simulink model "paper1"  (Simulink 6.0)
settings: Solver=ode45  StartTime=0.0  StopTime=30.0  RelTol=1e-3
values from neighbouring files (symbols this model uses):
  bp = 0.0    (= 0)    [paper1_data.m]
  bt = 0.8    [paper1_data.m]
  En = 1.0    (= 1)    [paper1_data.m]
  Eqh = 0.5    [paper1_data.m]
  Ey = 1.0    (= 1)    [paper1_data.m]
  Ta = 5    [paper1_data.m]
  Td = 3.36    [paper1_data.m]
  Ti = 0.05    [paper1_data.m]
  Tn = 0.0    (= 0)    [paper1_data.m]
  Tw = 1.0    (= 1)    [paper1_data.m]
  Ty = 0.2    [paper1_data.m]
settings Model: LastModifiedBy=Administrator

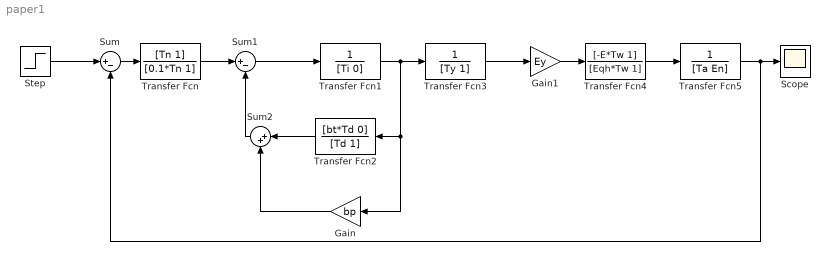
== system paper1 ==
  Gain : Gain  Orientation=left  Gain=bp
  Gain1 : Gain  Gain=Ey
  Scope : Scope
  Step : Step  SampleTime=0
  Sum : Sum  Inputs=|+-
  Sum1 : Sum  Inputs=|+-
  Sum2 : Sum  Orientation=left  Inputs=|++
  Transfer Fcn : TransferFcn  Numerator=[Tn 1]  Denominator=[0.1*Tn 1]
  Transfer Fcn1 : TransferFcn  Denominator=[Ti 0]
  Transfer Fcn2 : TransferFcn  Orientation=left  Numerator=[bt*Td 0]  Denominator=[Td 1]
  Transfer Fcn3 : TransferFcn  Denominator=[Ty 1]
  Transfer Fcn4 : TransferFcn  Numerator=[-E*Tw 1]  Denominator=[Eqh*Tw 1]
  Transfer Fcn5 : TransferFcn  Denominator=[Ta En]
  wires:
  Step/1 -> Sum/1
  Sum/1 -> Transfer Fcn/1
  Transfer Fcn/1 -> Sum1/1
  Transfer Fcn1/1 -> Transfer Fcn3/1, Transfer Fcn2/1, Gain/1
  Transfer Fcn3/1 -> Gain1/1
  Gain1/1 -> Transfer Fcn4/1
  Transfer Fcn4/1 -> Transfer Fcn5/1
  Transfer Fcn5/1 -> Scope/1, Sum/2
  Sum1/1 -> Transfer Fcn1/1
  Gain/1 -> Sum2/2
  Transfer Fcn2/1 -> Sum2/1
  Sum2/1 -> Sum1/2
